simulink model "Subsystem"  (R2020b)
settings: Solver=VariableStepAuto  StartTime=0.0  StopTime=10.0  RelTol=1e-3
settings Model: Creator=dell  LastModifiedBy=dell
settings DataIOCC: SaveOutput=off  SaveTime=off

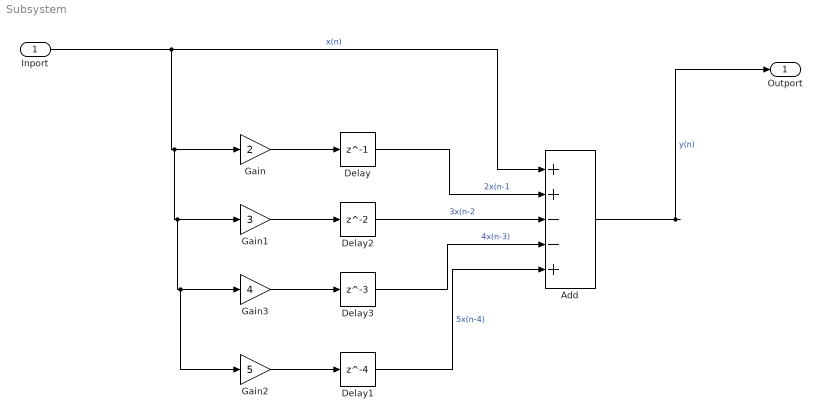
== system Subsystem ==
  Inport : Inport
  Add : Sum  Inputs=++--+
  Delay : Delay  DelayLength=1
  Delay1 : Delay  DelayLength=4
  Delay2 : Delay
  Delay3 : Delay  DelayLength=3
  Gain : Gain  Gain=2
  Gain1 : Gain  Gain=3
  Gain2 : Gain  Gain=5
  Gain3 : Gain  Gain=4
  Outport : Outport
  wires:
  Gain/1 -> Delay/1
  Inport/1 -> Add/1, Gain/1, Gain1/1, Gain3/1, Gain2/1  "x(n)"
  Gain3/1 -> Delay3/1
  Delay2/1 -> Add/3  "3x(n-2"
  Delay1/1 -> Add/5  "5x(n-4)"
  Gain2/1 -> Delay1/1
  Delay3/1 -> Add/4  "4x(n-3)"
  Gain1/1 -> Delay2/1
  Add/1 -> Outport/1  "y(n)"
  Delay/1 -> Add/2  "2x(n-1"
